simulink model "eoc_2"  (R2018b)
settings: Solver=VariableStepAuto  StartTime=0.0  StopTime=10.0  RelTol=1e-3
settings Model: Creator=nharada  LastModifiedBy=nharada

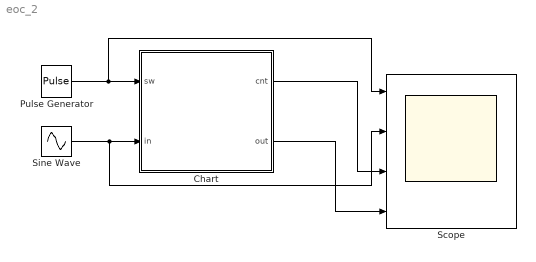
== system eoc_2 ==
  Chart : Stateflow chart  TreatAsAtomicUnit=on
  Pulse Generator : DiscretePulseGenerator  PulseType=Time based  PulseWidth=70  PhaseDelay=0.01
  Scope : Scope  NumInputPorts=4
  Sine Wave : Sin  Frequency=10  SampleTime=0.01
  wires:
  Pulse Generator/1 -> Chart/1(sw), Scope/1
  Sine Wave/1 -> Scope/2, Chart/2(in)
  Chart/1(cnt) -> Scope/3
  Chart/2(out) -> Scope/4

== stateflow chart eoc_2/Chart ==
  state off
    en,du:
    out = 0;
  state st1
    entry:
    cnt = 0;
    out = 0;
  state on
    entry:
    cnt = cnt + 1;
    en,du:
    out = in;
  st1 -> off : [sw == 0]
  off -> on : [sw == 1]
  (default) -> st1
  on -> off : [sw==0]
  data: sw input; in input; cnt output; out output
